simulink model "auto_pilot_upl_20240129"  (R2022b)
settings: Solver=FixedStepAuto  StartTime=0.0  StopTime=Inf  FixedStep=0.001  RelTol=1e-3  EnableMultiTasking=on
InitFcn:
  | clear mex
model workspace (MAT data in the model file):
  worldsim_instance : object (value not decoded)
values from neighbouring files (symbols this model uses):
  ACC_Adaptive_D = 0    [AutoPilot_parameters.m]    (also in ap_ini_param.mat; ap_initialModel.sldd = 0.0)
  ACC_Adaptive_I = 0    [AutoPilot_parameters.m]    (also in ap_ini_param.mat; ap_initialModel.sldd = 0.0)
  ACC_Adaptive_P = [5 7.5]    [AutoPilot_parameters.m]    (also in ap_ini_param.mat; ap_initialModel.sldd = 5.0 7.5)
  ACC_Classic_I = 5    [AutoPilot_parameters.m]    (also in ap_ini_param.mat; ap_initialModel.sldd = 5.0)
  ACC_Classic_P = 15    [AutoPilot_parameters.m]    (also in ap_ini_param.mat; ap_initialModel.sldd = 15.0)
  ACC_MaxBrake = 50    [AutoPilot_parameters.m]    (also in ap_ini_param.mat; ap_initialModel.sldd = 50.0)
  ACC_MaxThrottle = 130    [AutoPilot_parameters.m]    (also in ap_ini_param.mat = 80; ap_initialModel.sldd = 130.0)
  ACC_Module_Activity_Flag = 1    [AutoPilot_parameters.m]    (also in ap_ini_param.mat; ap_initialModel.sldd = 1.0)
  ACC_Ready_Speed = 30    [AutoPilot_parameters.m]    (also in ap_ini_param.mat; ap_initialModel.sldd = 30.0)
  ACC_SensorMaxDistance = 250    [AutoPilot_parameters.m]    (also in ap_ini_param.mat = 120; ap_initialModel.sldd = 250.0)
  ACC_Speed_Distance_control = 3    [AutoPilot_parameters.m]    (also in ap_ini_param.mat; ap_initialModel.sldd = 3.0)
  ACC_Speed_Distance_Gain = [0.1 0.15 0.2 0.25]    [AutoPilot_parameters.m]    (also in ap_ini_param.mat; ap_initialModel.sldd = 0.1 0.15 0.2 0.25)
  ADAS_Control_Mode = 1    [AutoPilot_parameters.m]    (also in ap_ini_param.mat; ap_initialModel.sldd = 1.0)
  AEB_Alarm_Freq = 5    [AutoPilot_parameters.m]    (also in ap_ini_param.mat; ap_initialModel.sldd = 5.0)
  AEB_Distance_To_Collision_Brake = 5    [AutoPilot_parameters.m]    (also in ap_ini_param.mat; ap_initialModel.sldd = 5.0)
  AEB_Freq_Hz = Sensor_Freq_worldsim/2    (= 25)    [AutoPilot_parameters.m]    (also in ap_ini_param.mat; ap_initialModel.sldd = 25.0)
  AEB_Gain = [1 1]    [AutoPilot_parameters.m]    (also in ap_ini_param.mat; ap_initialModel.sldd = 1.0 1.0)
  AEB_Gain_set = 60    [AutoPilot_parameters.m]    (also in ap_ini_param.mat; ap_initialModel.sldd = 60.0)
  AEB_Gain_set_mult = 0.03    [AutoPilot_parameters.m]    (also in ap_ini_param.mat; ap_initialModel.sldd)
  AEB_Max_Decel = [8 15]    [AutoPilot_parameters.m]    (also in ap_ini_param.mat; ap_initialModel.sldd = 8.0 15.0)
  AEB_Max_Speed = 150    [AutoPilot_parameters.m]    (also in ap_ini_param.mat = 100; ap_initialModel.sldd = 150.0)
  AEB_Min_Distance_at_Stop = 1    [AutoPilot_parameters.m]    (also in ap_ini_param.mat; ap_initialModel.sldd = 1.0)
  AEB_Module_Activity_Flag = 1    [AutoPilot_parameters.m]    (also in ap_ini_param.mat; ap_initialModel.sldd = 1.0)
  AEB_Pedestrian_type = 68    [AutoPilot_parameters.m]    (also in ap_ini_param.mat; ap_initialModel.sldd = 68.0)
  AEB_Steer_Max = 180    [AutoPilot_parameters.m]    (also in ap_ini_param.mat; ap_initialModel.sldd = 180.0)
  AP_Activity_Flag = 1    [AutoPilot_parameters.m]    (also in ap_ini_param.mat; ap_initialModel.sldd = 1.0)
  AP_D = [0.3 0.3]    [AutoPilot_parameters.m]    (also in ap_ini_param.mat; ap_initialModel.sldd = 0.3 0.3)
  AP_Dyn_Rate_Limiter_Gain = 0.1    [AutoPilot_parameters.m]    (also in ap_ini_param.mat; ap_initialModel.sldd)
  AP_Dyn_Rate_Limiter_Power = 10    [AutoPilot_parameters.m]    (also in ap_ini_param.mat; ap_initialModel.sldd = 10.0)
  AP_Error_Max = 3    [AutoPilot_parameters.m]    (also in ap_ini_param.mat; ap_initialModel.sldd = 3.0)
  AP_Freq_Hz = Sensor_Freq_worldsim    (= 50)    [AutoPilot_parameters.m]    (also in ap_ini_param.mat; ap_initialModel.sldd = 50.0)
  AP_I = [0.05 0.05]    [AutoPilot_parameters.m]    (also in ap_ini_param.mat; ap_initialModel.sldd = 0.05 0.05)
  AP_Max_Error_dydt_Disable = 0.5    [AutoPilot_parameters.m]    (also in ap_ini_param.mat; ap_initialModel.sldd)
  AP_On_Request_Time = 0.01    [AutoPilot_parameters.m]    (also in ap_ini_param.mat; ap_initialModel.sldd)
  AP_P = [0.2 0.2]    [AutoPilot_parameters.m]    (also in ap_ini_param.mat; ap_initialModel.sldd = 0.2 0.2)
  AP_Steer_Error_Max = 0.7    [AutoPilot_parameters.m]    (also in ap_ini_param.mat; ap_initialModel.sldd)
  AP_Steer_Rate_Max_radps = 1    [AutoPilot_parameters.m]    (also in ap_ini_param.mat; ap_initialModel.sldd = 1.0)
  AP_Transition_Rate = 0.5    [AutoPilot_parameters.m]    (also in ap_ini_param.mat; ap_initialModel.sldd)
  butter_a = [1 -1.9911142922 0.991153595869]    [ap_ini_param.mat]    (also in ap_initialModel.sldd = 1.0 -1.9911142922016536 0.99115359586893548)
  butter_b = [9.82591682048e-06 1.9651833641e-05 9.82591682048e-06]    [ap_ini_param.mat]    (also in ap_initialModel.sldd = 9.825916820482009E-6 1.9651833640964018E-5 9.825916820482009)
  Lane_Width = 3.7    [AutoPilot_parameters.m]    (also in ap_ini_param.mat; ap_initialModel.sldd)
  No_Target_Display_Value = 0    [AutoPilot_parameters.m]    (also in ap_ini_param.mat; ap_initialModel.sldd = 0.0)
  radar_source = 2    [AutoPilot_parameters.m]    (also in ap_ini_param.mat; ap_initialModel.sldd = 2.0)
  Sensor_Freq_worldsim = 50    [AutoPilot_parameters.m]    (also in ap_ini_param.mat; ap_initialModel.sldd = 50.0; launcher.m)
  stop_number_collisions = 10.0    [ap_initialModel.sldd]    (also in launcher.m = 10)
  stop_speed = 0.001    [ap_initialModel.sldd]    (also in launcher.m)
  stop_time = 12.0    [ap_initialModel.sldd]    (also in launcher.m = 12)
  vehicle_width = 2.2    [AutoPilot_parameters.m]    (also in ap_ini_param.mat = 1.86; ap_initialModel.sldd)
undefined symbols (not defined in the file or in its folder): blockPlatform, light_brake_center, light_brake_left, light_brake_right
libraries: simulink x82, simwbSfunlib x32, viworldsim_lib x5, slpidlib x4, simwbUDPBlocklib x1
(part 2 of 4)

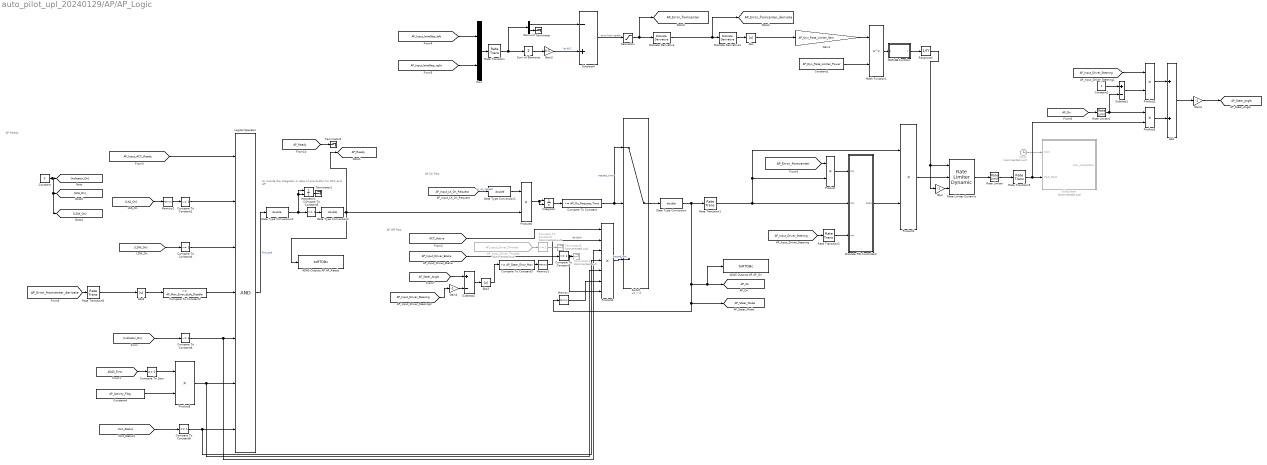
== system auto_pilot_upl_20240129/AP/AP_Logic ==
  note: to include the integrator in case of one button
      | for ACC and AP
  note: AP Off Req
  note: AP Ready
  note: AP On Req
  ADAS.Outputs.AP.AP_On : simwbSfunlib/toRTDBc  stringBlock=off  varName=ADAS.Outputs.AP.AP_On  sigDim=[1 1]  sigType=double  sampleTime=[-1 0]  maxBuffSize=1024  busName=nobus  defaultValue=0  defaultString=simwbout  hasMapping=0  ptrName=ADAS_Outputs_AP_AP_Ready  enumOrAlias=nothing
      settings: SourceProductName=SimWB MLToolkit
  ADAS.Outputs.AP.AP_Ready : simwbSfunlib/toRTDBc  stringBlock=off  varName=ADAS.Outputs.AP.AP_Ready  sigDim=[1 1]  sigType=double  sampleTime=[-1 0]  maxBuffSize=1024  busName=nobus  defaultValue=0  defaultString=simwbout  hasMapping=0  ptrName=varName  enumOrAlias=nothing
      settings: SourceProductName=SimWB MLToolkit
  AP_Input_Driver_Throttle : From  Commented=on  GotoTag=AP_Input_Driver_Throttle  TagVisibility=global
  Abs : Abs  SaturateOnIntegerOverflow=off
  Abs2 : Abs  SaturateOnIntegerOverflow=off
  Abs3 : Abs  SaturateOnIntegerOverflow=off
  Add : Sum
  Clock : Clock  Commented=on
  Compare To Constant : simulink/Logic and Bit Operations/Compare To Constant  relop=>=  const=AP_On_Request_Time  OutDataTypeStr=boolean
  Compare To Constant1 : simulink/Logic and Bit Operations/Compare To Constant  relop=~=  const=1  OutDataTypeStr=boolean
  Compare To Constant2 : simulink/Logic and Bit Operations/Compare To Constant  relop=<=  const=AP_Max_Error_dydt_Disable  OutDataTypeStr=boolean
  Compare To Constant3 : simulink/Logic and Bit Operations/Compare To Constant  relop=<=  const=AP_Steer_Error_Max  OutDataTypeStr=boolean
  Compare To Constant4 : simulink/Logic and Bit Operations/Compare To Constant  relop=~=  const=1  OutDataTypeStr=boolean
  Compare To Constant5 : simulink/Logic and Bit Operations/Compare To Constant  relop=>=  const=1  OutDataTypeStr=boolean
  Compare To Constant6 : simulink/Logic and Bit Operations/Compare To Constant  relop=~=  const=1  OutDataTypeStr=boolean
  Compare To Constant7 : simulink/Logic and Bit Operations/Compare To Constant  Commented=on  relop=<=  const=1  OutDataTypeStr=boolean
  Compare To Constant8 : simulink/Logic and Bit Operations/Compare To Constant  relop===  const=1  OutDataTypeStr=boolean
  Compare To Constant9 : simulink/Logic and Bit Operations/Compare To Constant  relop=<=  const=1  OutDataTypeStr=boolean
  Compare To Zero : simulink/Logic and Bit Operations/Compare To Zero  relop===  OutDataTypeStr=boolean
  Constant : Constant  Value=0
  Constant1 : Constant  Value=AP_Dyn_Rate_Limiter_Power
  Constant2 : Constant
  Constant4 : Constant  Value=AP_Activity_Flag
  Data Type Conversion{,1..3} (4 alike) : DataTypeConversion  OutDataTypeStr=double  SaturateOnIntegerOverflow=off  RndMeth=Floor
  Demux3 : Demux  Outputs=2
  Discrete Derivative : simulink/Discrete/Discrete Derivative  gainval=1.0  ICPrevScaledInput=0.0  OutMin=[]  OutMax=[]  OutDataType=fixdt(1, 16)  OutScaling=2^-10  DoSatur=off
  Discrete Derivative1 : simulink/Discrete/Discrete Derivative  gainval=1.0  ICPrevScaledInput=0.0  OutMin=[]  OutMax=[]  OutDataType=fixdt(1, 16)  OutScaling=2^-10  DoSatur=off
  Discrete PID Controller2 : Subsystem
  Gain : Gain  Gain=-1
  Gain1 : Gain  Gain=AP_Dyn_Rate_Limiter_Gain
  Gain2 : Gain  Gain=-1
  Gain3 : Gain  Gain=0.5
  Gain4 : Gain  Gain=-1
  Integrator : Integrator  ExternalReset=either
  Integrator1 : Integrator  ExternalReset=either
  Logical Operator : Logic  Inputs=7  AllPortsSameDT=off  OutDataTypeStr=boolean
  MATLAB Function : MATLAB Function  TreatAsAtomicUnit=on
  Math Function1 : Math  Operator=pow  SignedPower=on
  Memory : Memory
  Memory1 : Memory
  Memory2 : Memory
  Mux : Mux  Inputs=2
  Product{,1..3,5..6} (6 alike) : Product
  Product4 : Product  Inputs=7
  Rate Limiter : RateLimiter  RisingSlewLimit=AP_Steer_Rate_Max_radps  FallingSlewLimit=-AP_Steer_Rate_Max_radps  SampleTimeMode=inherited
  Rate Limiter Dynamic : simulink/Discontinuities/Rate Limiter Dynamic
  Rate Limiter1 : RateLimiter  RisingSlewLimit=AP_Transition_Rate  FallingSlewLimit=-AP_Transition_Rate  SampleTimeMode=inherited
  Rate Transition : RateTransition  OutPortSampleTime=1/AP_Freq_Hz
  Rate Transition1 : RateTransition  OutPortSampleTime=1/AP_Freq_Hz
  Rate Transition2 : RateTransition  OutPortSampleTime=1/AP_Freq_Hz
  Rate Transition5 : RateTransition  OutPortSampleTime=1/1000
  Rate Transition8 : RateTransition  OutPortSampleTime=1/1000
  Reciprocal : Product  Inputs=/  RndMeth=Zero  SaturateOnIntegerOverflow=on
  Saturation : Saturate  UpperLimit=AP_Error_Max  LowerLimit=-AP_Error_Max
  Subsystem : Subsystem  Commented=on
  Subtract1 : Sum  Inputs=+-
  Subtract2 : Sum  Inputs=+-
  Subtract4 : Sum  Inputs=-+
  Sum of Elements : Sum  Inputs=+
  Switch : Switch  Criteria=u2 > Threshold  SaturateOnIntegerOverflow=off  InputSameDT=off
  Terminator : Terminator
  Terminator1 : Terminator
  Terminator2 : Terminator
  Terminator3 : Terminator  Commented=on
  Terminator4 : Terminator  Commented=on
  tag scope: AP_Error_fromcenter=global, AP_Error_fromcenter_derivate=global, AP_On=global, AP_Ready=global, AP_Steer_Angle=global, AP_Steer_Mode=global
  wires:
  Discrete Derivative/1 -> Discrete Derivative1/1, [AP_Error_fromcenter_derivate]
  Rate Transition1/1 -> Discrete PID Controller2/2(In2), Product1/1, Product/2
  Constant1/1 -> Math Function1/2
  Math Function1/1 -> MATLAB Function/1(u)
  Discrete Derivative1/1 -> Abs/1
  Gain1/1 -> Math Function1/1
  Reciprocal/1 -> Gain/1, Rate Limiter Dynamic/1
  Abs/1 -> Gain1/1
  Gain/1 -> Rate Limiter Dynamic/3
  Rate Limiter Dynamic/1 -> Rate Limiter/1
  Product1/1 -> Rate Limiter Dynamic/2
  Clock/1 -> Subsystem/1(Clock)
  Rate Limiter/1 -> Rate Transition5/1
  Saturation/1 -> [AP_Error_fromcenter], Discrete Derivative/1
  Constant2/1 -> Subtract1/1
  Subtract1/1 -> Product2/2
  Rate Limiter1/1 -> Subtract1/2, Product3/1
  Product2/1 -> Add/1
  Product3/1 -> Add/2
  Add/1 -> Gain2/1
  Subtract2/1 -> Abs3/1
  [AP_Input_LK_On_Request] -> Data Type Conversion1/1  "LK_on_request"
  Switch/1 -> Data Type Conversion/1
  Product4/1 -> Switch/3  "second_and"
  Data Type Conversion/1 -> Memory/1, [AP_Steer_Mode], ADAS.Outputs.AP.AP_On/1, [AP_On], Rate Transition1/1
  Data Type Conversion1/1 -> Product6/1
  Rate Transition8/1 -> Abs2/1
  Abs2/1 -> Compare To Constant2/1
  Compare To Constant2/1 -> Logical Operator/4
  Abs3/1 -> Compare To Constant3/1
  Compare To Constant3/1 -> Memory1/1
  [LDW_On] -> Compare To Constant4/1
  Compare To Constant4/1 -> Logical Operator/3
  Memory1/1 -> Product4/2  "de-latch"
  [LKA_On] -> Memory2/1
  Memory2/1 -> Compare To Constant1/1
  Integrator/1 -> Compare To Constant/1
  Product6/1 -> Integrator/1, Integrator/2
  Compare To Constant1/1 -> Logical Operator/2
  Logical Operator/1 -> Data Type Conversion3/1  "first_and"
  Compare To Constant/1 -> Switch/1, Switch/2  "request_time"
  Data Type Conversion2/1 -> Product6/2, ADAS.Outputs.AP.AP_Ready/1, [AP_Ready]
  Data Type Conversion3/1 -> Integrator1/1, Integrator1/2, Compare To Constant5/1
  Compare To Constant5/1 -> Data Type Conversion2/1
  [Indicator_On] -> Compare To Constant6/1
  Compare To Constant6/1 -> Product4/3, Logical Operator/5
  Rate Transition/1 -> Demux3/1, Sum of Elements/1
  Sum of Elements/1 -> Gain3/1
  Gain3/1 -> Subtract4/2  "(a+b)/2"
  Demux3/2 -> Terminator/1
  Demux3/1 -> Subtract4/1
  Subtract4/1 -> Saturation/1  "error from center"
  [ADAS_Error] -> Compare To Zero/1
  Constant4/1 -> Product5/2
  Compare To Zero/1 -> Product5/1
  Product5/1 -> Logical Operator/6, Product4/5
  [Vicrt_Status] -> Compare To Constant8/1
  Compare To Constant8/1 -> Product4/4, Logical Operator/7
  [AP_Input_Driver_Steering] -> Rate Transition2/1
  Product/1 -> Discrete PID Controller2/1(In1)
  Rate Transition2/1 -> Discrete PID Controller2/3(In4)
  Discrete PID Controller2/1(Out1) -> Product1/2
  Rate Transition5/1 -> Product3/2, Subsystem/2(Input_Signal)
  [AP_Input_ACC_Ready] -> Logical Operator/1
  AP_Input_Driver_Throttle/1 -> Compare To Constant7/1
  Compare To Constant9/1 -> Product4/7, Terminator4/1
  [AP_Input_Driver_Brake] -> Compare To Constant9/1
  Compare To Constant7/1 -> Terminator3/1
  [ACC_Active] -> Product4/1
  Integrator1/1 -> Terminator1/1
  Mux/1 -> Rate Transition/1
  [AP_Input_laneGap_left] -> Mux/1
  [AP_Input_laneGap_right] -> Mux/2
  [AP_Error_fromcenter_derivate] -> Rate Transition8/1
  [AP_Input_Driver_Steering] -> Product2/1
  [AP_Input_Driver_Steering] -> Gain4/1
  [AP_Steer_Angle] -> Subtract2/1
  [AP_On] -> Rate Limiter1/1
  [AP_Error_fromcenter] -> Product/1
  Gain2/1 -> [AP_Steer_Angle]
  Memory/1 -> Product4/6
  Gain4/1 -> Subtract2/2
  Constant/1 -> [LDW_On], [LKA_On], [Indicator_On]
  [AP_Ready] -> Terminator2/1
  MATLAB Function/1(y) -> Reciprocal/1

== system auto_pilot_upl_20240129/AP/AP_Outputs ==
  Terminator : Terminator
  tag scope: AP_Output_Steer_Angle=global, AP_Output_Steer_Torque=global
  wires:
  [AP_Steer_Mode] -> [AP_Output_Steer_Torque]
  [AP_Steer_Angle] -> [AP_Output_Steer_Angle]
  [AP_Output_Steer_Torque] -> Terminator/1

== system auto_pilot_upl_20240129/INPUT/Inputs for CRT ==
  Clutch_manager : Subsystem
  Constant : Constant  Value=0
  Constant1 : Constant
  tag scope: brake_demand=global, clutch_demand=global, gear_demand=global, steering_angle_demand=global, steering_torque_demand=global, throttle_demand=global
  wires:
  [ACC_Output_Brake] -> [brake_demand]
  Constant/1 -> [steering_torque_demand]
  [AP_Output_Steer_Angle] -> [steering_angle_demand]
  Clutch_manager/1(clutch) -> [clutch_demand]
  [ACC_Output_Throttle] -> [throttle_demand]
  [ACC_Output_Throttle] -> Clutch_manager/1(throttle)
  Constant1/1 -> [gear_demand]

== system auto_pilot_upl_20240129/OUTPUT/VI-CarRealTime_Outputs ==
  Gain : Gain  Gain=1/2
  Log_bus : BusSelector  OutputSignals=VI_CarRealTime:Outputs:chassis_velocities:longitudinal,VI_CarRealTime:Outputs:driver_demands:steering,VI_CarRealTime:Outputs:Wheel:Spindle_Steer:L1,VI_CarRealTime:Outputs:Wheel:Spindle_Steer:R1,VI_CarRealTime:Outputs:driver_demands:throttle,VI_CarRealTime:Outputs:driver_demands:brake,VI_CarRealTime:Outputs:chassis_accelerations:longitudinal,VI_CarRealTime:Outputs:chassis_accelerations:lateral,VI_CarRealTime:Outputs:Steering_System:DriveSim_Steering_Feedback_Torque  OutputAsBus=on
  Scope : Scope  NumInputPorts=2
  Sum : Sum
  Terminator : Terminator
  internal_bus : BusSelector  OutputSignals=VI_CarRealTime:Outputs:chassis_velocities:longitudinal,VI_CarRealTime:Outputs:driver_demands:steering,VI_CarRealTime:Outputs:Wheel:Spindle_Steer:L1,VI_CarRealTime:Outputs:Wheel:Spindle_Steer:R1,VI_CarRealTime:Outputs:driver_demands:throttle,VI_CarRealTime:Outputs:driver_demands:brake,VI_CarRealTime:Outputs:chassis_accelerations:longitudinal,VI_CarRealTime:Outputs:chassis_accelerations:lateral,VI_CarRealTime:Outputs:Steering_System:DriveSim_Steering_Feedback_Torque
  tag scope: Driver_Brake=global, Driver_Steering=global, Driver_Throttle=global, Front_Axle_Steer=global, Lateral_Accelerations=global, Longitudinal_Accelerations=global, Steering_feedback_torque=global, Vehicle_Speed=global
  wires:
  internal_bus/9 -> [Steering_feedback_torque]  "<VI_CarRealTime:Outputs:Steering_System:DriveSim_Steering_Feedback_Torque>"
  internal_bus/8 -> [Lateral_Accelerations]  "<VI_CarRealTime:Outputs:chassis_accelerations:lateral>"
  internal_bus/7 -> [Longitudinal_Accelerations]  "<VI_CarRealTime:Outputs:chassis_accelerations:longitudinal>"
  internal_bus/6 -> [Driver_Brake]  "<VI_CarRealTime:Outputs:driver_demands:brake>"
  internal_bus/5 -> [Driver_Throttle]  "<VI_CarRealTime:Outputs:driver_demands:throttle>"
  Gain/1 -> [Front_Axle_Steer]
  Sum/1 -> Gain/1
  internal_bus/4 -> Sum/2  "<VI_CarRealTime:Outputs:Wheel:Spindle_Steer:R1>"
  internal_bus/3 -> Sum/1  "<VI_CarRealTime:Outputs:Wheel:Spindle_Steer:L1>"
  [Vehicle_outputs] -> internal_bus/1, Log_bus/1
  internal_bus/2 -> [Driver_Steering], Scope/2  "<VI_CarRealTime:Outputs:driver_demands:steering>"
  Log_bus/1 -> Terminator/1  "VI_CarRealTime_selection"
  internal_bus/1 -> [Vehicle_Speed], Scope/1  "<VI_CarRealTime:Outputs:chassis_velocities:longitudinal>"

== system auto_pilot_upl_20240129/OUTPUT/VI-CarRealTime_Outputs2 ==
  Constant : Constant  Value=0
  Gain : Gain  Gain=1/2
  Log_Bus_Creator : BusCreator  Inputs=9
  Log_bus : BusSelector  OutputSignals=VI_CarRealTime:Outputs:chassis_velocities:longitudinal,VI_CarRealTime:Outputs:driver_demands:steering,VI_CarRealTime:Outputs:Wheel:Spindle_Steer:L1,VI_CarRealTime:Outputs:Wheel:Spindle_Steer:R1,VI_CarRealTime:Outputs:driver_demands:throttle,VI_CarRealTime:Outputs:driver_demands:brake,VI_CarRealTime:Outputs:chassis_accelerations:longitudinal,VI_CarRealTime:Outputs:chassis_accelerations:lateral,VI_CarRealTime:Outputs:Steering_System:DriveSim_Steering_Feedback_Torque  OutputAsBus=on
  Scope : Scope  NumInputPorts=2
  Sum : Sum
  Terminator : Terminator
  Terminator1 : Terminator
  VI_CarRealTime.Outputs.Steering_System.DriveSim_Steering_Feedback_Torque : simwbSfunlib/fromRTDBm  varName=VI_CarRealTime.Outputs.Steering_System.DriveSim_Steering_Feedback_Torque  sigDim=[1 1]  sigType=double  sampleTime=[-1 0]  defaultValue=0  hasMapping=0  ptrName=VI_CarRealTime_Outputs_chassis_accelerations_lateral  enumOrAlias=nothing
      settings: SourceProductName=SimWB MLToolkit
  VI_CarRealTime.Outputs.Wheel.Spindle_Steer.L1 : simwbSfunlib/fromRTDBm  varName=VI_CarRealTime.Outputs.Wheel.Spindle_Steer.L1  sigDim=[1 1]  sigType=double  sampleTime=[-1 0]  defaultValue=0  hasMapping=0  ptrName=VI_CarRealTime_Outputs_Wheel_Spindle_Steer_L1  enumOrAlias=nothing
      settings: SourceProductName=SimWB MLToolkit
  VI_CarRealTime.Outputs.Wheel.Spindle_Steer.R1 : simwbSfunlib/fromRTDBm  varName=VI_CarRealTime.Outputs.Wheel.Spindle_Steer.R1  sigDim=[1 1]  sigType=double  sampleTime=[-1 0]  defaultValue=0  hasMapping=0  ptrName=VI_CarRealTime_Outputs_Wheel_Spindle_Steer_R1  enumOrAlias=nothing
      settings: SourceProductName=SimWB MLToolkit
  VI_CarRealTime.Outputs.chassis_accelerations.lateral : simwbSfunlib/fromRTDBm  varName=VI_CarRealTime.Outputs.chassis_accelerations.lateral  sigDim=[1 1]  sigType=double  sampleTime=[-1 0]  defaultValue=0  hasMapping=0  ptrName=VI_CarRealTime_Outputs_chassis_accelerations_longitudinal  enumOrAlias=nothing
      settings: SourceProductName=SimWB MLToolkit
  VI_CarRealTime.Outputs.chassis_accelerations.longitudinal : simwbSfunlib/fromRTDBm  varName=VI_CarRealTime.Outputs.chassis_accelerations.longitudinal  sigDim=[1 1]  sigType=double  sampleTime=[-1 0]  defaultValue=0  hasMapping=0  ptrName=VI_CarRealTime_Outputs_chassis_velocities_longitudinal  enumOrAlias=nothing
      settings: SourceProductName=SimWB MLToolkit
  VI_CarRealTime.Outputs.chassis_velocities.longitudinal : simwbSfunlib/fromRTDBm  varName=VI_CarRealTime.Outputs.chassis_velocities.longitudinal  sigDim=[1 1]  sigType=double  sampleTime=[-1 0]  defaultValue=0  hasMapping=0  ptrName=VI_CarRealTime_Outputs_chassis_velocities_longitudinal  enumOrAlias=nothing
      settings: SourceProductName=SimWB MLToolkit
  VI_CarRealTime.Outputs.driver_demands.brake : simwbSfunlib/fromRTDBm  varName=VI_CarRealTime.Outputs.driver_demands.brake  sigDim=[1 1]  sigType=double  sampleTime=[-1 0]  defaultValue=0  hasMapping=0  ptrName=VI_CarRealTime_Outputs_driver_demands_throttle  enumOrAlias=nothing
      settings: SourceProductName=SimWB MLToolkit
  VI_CarRealTime.Outputs.driver_demands.steering : simwbSfunlib/fromRTDBm  varName=VI_CarRealTime.Outputs.driver_demands.steering  sigDim=[1 1]  sigType=double  sampleTime=[-1 0]  defaultValue=0  hasMapping=0  ptrName=VI_CarRealTime_Outputs_chassis_velocities_longitudinal  enumOrAlias=nothing
      settings: SourceProductName=SimWB MLToolkit
  VI_CarRealTime.Outputs.driver_demands.throttle : simwbSfunlib/fromRTDBm  varName=VI_CarRealTime.Outputs.driver_demands.throttle  sigDim=[1 1]  sigType=double  sampleTime=[-1 0]  defaultValue=0  hasMapping=0  ptrName=VI_CarRealTime_Outputs_driver_demands_steering  enumOrAlias=nothing
      settings: SourceProductName=SimWB MLToolkit
  tag scope: Driver_Brake=global, Driver_Steering=global, Driver_Throttle=global, Front_Axle_Steer=global, Lateral_Accelerations=global, Longitudinal_Accelerations=global, Steering_feedback_torque=global, Vehicle_Speed=global
  wires:
  ? -> Scope/1, [Vehicle_Speed]
  Log_bus/1 -> Terminator/1  "VI_CarRealTime_selection"
  ? -> Scope/2, [Driver_Steering]
  ? -> Sum/1
  ? -> Sum/2
  Sum/1 -> Gain/1
  Gain/1 -> [Front_Axle_Steer]
  ? -> [Driver_Throttle]
  Constant/1 -> [Driver_Brake]
  ? -> Terminator1/1
  ? -> [Longitudinal_Accelerations]
  ? -> [Lateral_Accelerations]
  ? -> [Steering_feedback_torque]
  VI_CarRealTime.Outputs.driver_demands.brake/1 -> Log_Bus_Creator/6  "VI_CarRealTime.Outputs.driver_demands.brake"
  VI_CarRealTime.Outputs.Wheel.Spindle_Steer.L1/1 -> Log_Bus_Creator/3  "VI_CarRealTime.Outputs.Wheel.Spindle_Steer.L1"
  VI_CarRealTime.Outputs.chassis_accelerations.lateral/1 -> Log_Bus_Creator/8  "VI_CarRealTime.Outputs.chassis_accelerations.lateral"
  VI_CarRealTime.Outputs.Steering_System.DriveSim_Steering_Feedback_Torque/1 -> Log_Bus_Creator/9  "VI_CarRealTime.Outputs.Steering_System.DriveSim_Steering_Feedback_Torque"
  VI_CarRealTime.Outputs.chassis_accelerations.longitudinal/1 -> Log_Bus_Creator/7  "VI_CarRealTime.Outputs.chassis_accelerations.longitudinal"
  VI_CarRealTime.Outputs.driver_demands.steering/1 -> Log_Bus_Creator/2  "VI_CarRealTime.Outputs.driver_demands.steering"
  VI_CarRealTime.Outputs.Wheel.Spindle_Steer.R1/1 -> Log_Bus_Creator/4  "VI_CarRealTime.Outputs.Wheel.Spindle_Steer.R1"
  VI_CarRealTime.Outputs.driver_demands.throttle/1 -> Log_Bus_Creator/5  "VI_CarRealTime.Outputs.driver_demands.throttle"
  VI_CarRealTime.Outputs.chassis_velocities.longitudinal/1 -> Log_Bus_Creator/1  "VI_CarRealTime.Outputs.chassis_velocities.longitudinal"
  Log_Bus_Creator/1 -> Log_bus/1

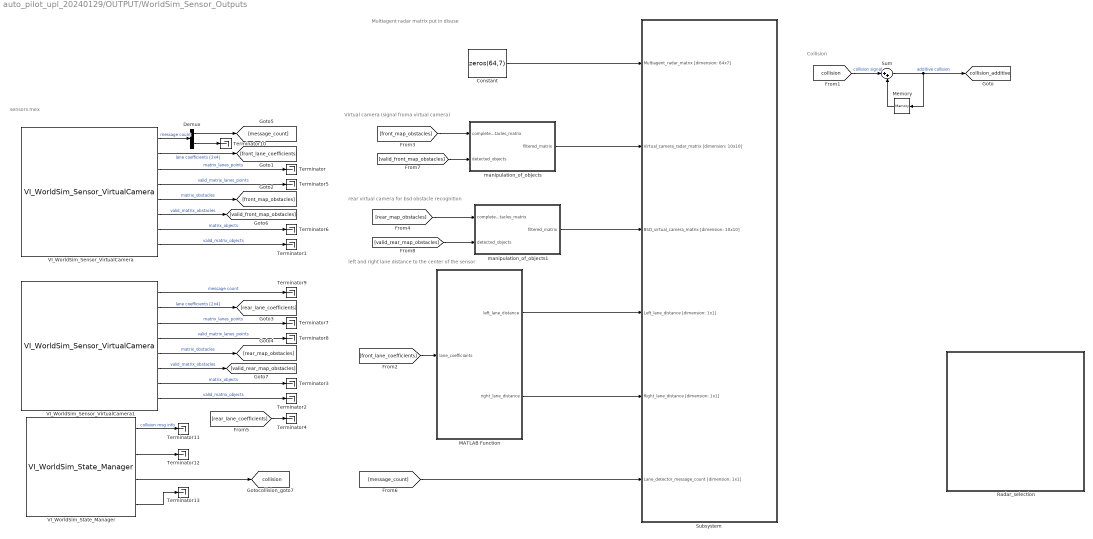
== system auto_pilot_upl_20240129/OUTPUT/WorldSim_Sensor_Outputs ==
  note: Collision
  note: left and right lane distance to the center of the sensor
  note: Virtual camera (signal froma virtual camera)
  note: Multiagent radar matrix
      | put in disuse
  note: rear virtual camera for bsd obstacle recognition
  note: sensors mex
  Constant : Constant  Value=zeros(64,7)
  Demux : Demux  Outputs=2
  MATLAB Function : MATLAB Function  TreatAsAtomicUnit=on
  Memory : Memory  InheritSampleTime=on
  Radar_selection : Subsystem
  Subsystem : Subsystem
  Sum : Sum  Inputs=|++
  Terminator{,1..13} (14 alike) : Terminator
  VI_WorldSim_Sensor_VirtualCamera : viworldsim_lib/VI-WorldSim Sensors/VI_WorldSim_Sensor_VirtualCamera  worldsim_endpoint_ip=worldsim_instance.endpoint_ip  worldsim_endpoint_port=worldsim_instance.endpoint_port  worldsim_car_name='ego'  worldsim_sensor_name='Front_VirtualCam'  max_lanes=10  max_obstacles=10  worldsim_verbose=off
  VI_WorldSim_Sensor_VirtualCamera1 : viworldsim_lib/VI-WorldSim Sensors/VI_WorldSim_Sensor_VirtualCamera  worldsim_endpoint_ip=worldsim_instance.endpoint_ip  worldsim_endpoint_port=worldsim_instance.endpoint_port  worldsim_car_name='ego'  worldsim_sensor_name='Rear_VirtualCam'  max_lanes=10  max_obstacles=10  worldsim_verbose=off
  VI_WorldSim_State_Manager : viworldsim_lib/VI-WorldSim Sensors/VI_WorldSim_State_Manager  worldsim_endpoint_ip=worldsim_instance.endpoint_ip  worldsim_endpoint_port=worldsim_instance.endpoint_port  worldsim_car_name='ego'  worldsim_verbose=off
  manipulation_of_objects : MATLAB Function  TreatAsAtomicUnit=on
  manipulation_of_objects1 : MATLAB Function  TreatAsAtomicUnit=on
  tag scope: collision=global, collision_additive=global
  wires:
  Sum/1 -> Memory/1, [collision_additive]  "additive collision"
  [collision] -> Sum/1  "collision signal"
  Memory/1 -> Sum/2
  MATLAB Function/1(left_lane_distance) -> Subsystem/4(Left_lane_distance [dimension: 1x1])
  [message_count] -> Subsystem/6(Lane_detector_message_count [dimension: 1x1])
  manipulation_of_objects1/1(filtered_matrix) -> Subsystem/3(BSD_virtual_camera_matrix [dimension: 10x10])
  manipulation_of_objects/1(filtered_matrix) -> Subsystem/2(Virtual_camera_radar_matrix [dimension: 10x10])
  Constant/1 -> Subsystem/1(Multiagent_radar_matrix [dimension: 64x7])
  [valid_rear_map_obstacles] -> manipulation_of_objects1/2(detected_objects)
  MATLAB Function/2(right_lane_distance) -> Subsystem/5(Right_lane_distance [dimension: 1x1])
  [front_lane_coefficients] -> MATLAB Function/1(lane_coefficiants)
  [rear_map_obstacles] -> manipulation_of_objects1/1(complete_obstacles_matrix)
  [valid_front_map_obstacles] -> manipulation_of_objects/2(detected_objects)
  [front_map_obstacles] -> manipulation_of_objects/1(complete_obstacles_matrix)
  VI_WorldSim_Sensor_VirtualCamera/1 -> Demux/1  "message count"
  VI_WorldSim_State_Manager/1 -> Terminator11/1  "collision msg info"
  VI_WorldSim_Sensor_VirtualCamera/8 -> Terminator1/1  "valid_matrix_objects"
  VI_WorldSim_Sensor_VirtualCamera/5 -> [front_map_obstacles]  "matrix_obstacles"
  VI_WorldSim_Sensor_VirtualCamera/4 -> Terminator5/1  "valid_matrix_lanes_points"
  VI_WorldSim_Sensor_VirtualCamera/6 -> [valid_front_map_obstacles]  "valid_matrix_obstacles"
  VI_WorldSim_Sensor_VirtualCamera1/2 -> [rear_lane_coefficients]  "lane coefficients [2x4]"
  VI_WorldSim_Sensor_VirtualCamera/3 -> Terminator/1  "matrix_lanes_points"
  VI_WorldSim_Sensor_VirtualCamera1/1 -> Terminator9/1  "message count"
  VI_WorldSim_Sensor_VirtualCamera1/7 -> Terminator3/1  "matrix_objects"
  VI_WorldSim_Sensor_VirtualCamera1/8 -> Terminator2/1  "valid_matrix_objects"
  VI_WorldSim_Sensor_VirtualCamera/7 -> Terminator6/1  "matrix_objects"
  VI_WorldSim_Sensor_VirtualCamera/2 -> [front_lane_coefficients]  "lane coefficients [2x4]"
  VI_WorldSim_Sensor_VirtualCamera1/4 -> Terminator8/1  "valid_matrix_lanes_points"
  VI_WorldSim_State_Manager/3 -> [collision]
  VI_WorldSim_Sensor_VirtualCamera1/3 -> Terminator7/1  "matrix_lanes_points"
  [rear_lane_coefficients] -> Terminator4/1
  Demux/2 -> Terminator10/1
  VI_WorldSim_Sensor_VirtualCamera1/5 -> [rear_map_obstacles]  "matrix_obstacles"
  VI_WorldSim_Sensor_VirtualCamera1/6 -> [valid_rear_map_obstacles]  "valid_matrix_obstacles"
  Demux/1 -> [message_count]
  VI_WorldSim_State_Manager/2 -> Terminator12/1
  VI_WorldSim_State_Manager/4 -> Terminator13/1

== system auto_pilot_upl_20240129/OUTPUT/rough data reporting ==
  Cast To Double : DataTypeConversion  OutDataTypeStr=double  SaturateOnIntegerOverflow=off  RndMeth=Floor
  Cast To Double1 : DataTypeConversion  OutDataTypeStr=double  SaturateOnIntegerOverflow=off  RndMeth=Floor
  Clock : Clock
  Compare To Constant : simulink/Logic and Bit Operations/Compare To Constant  relop=<=  const=0.0  OutDataTypeStr=boolean
  Compare To Constant1 : simulink/Logic and Bit Operations/Compare To Constant  relop=<=  const=0.0  OutDataTypeStr=boolean
  Compare To Constant2 : simulink/Logic and Bit Operations/Compare To Constant  relop=>  const=0.1  OutDataTypeStr=boolean
  Constant : Constant  Value=0
  Mux : Mux  Inputs=2
  Product : Product
  Scope LDW_Steering_Torque_in_out : Scope
  Sum1 : Sum
  To Workspace : ToWorkspace  VariableName=number_collision  SampleTime=-1
      settings: Save2DSignal=2-D array (concatenate along first dimension)
  To Workspace1 : ToWorkspace  VariableName=longitudinal_accelerations  SampleTime=-1
      settings: Save2DSignal=2-D array (concatenate along first dimension)
  To Workspace2 : ToWorkspace  VariableName=lateral_accelerations  SampleTime=-1
      settings: Save2DSignal=2-D array (concatenate along first dimension)
  To Workspace3 : ToWorkspace  VariableName=crossed_lanes  SampleTime=-1
      settings: Save2DSignal=2-D array (concatenate along first dimension)
  wires:
  Clock/1 -> Compare To Constant2/1
  Compare To Constant1/1 -> Cast To Double1/1
  [Lateral_Accelerations] -> To Workspace2/1
  [LaneGap_right_ws] -> Compare To Constant1/1
  Cast To Double/1 -> Sum1/1
  Compare To Constant2/1 -> Product/2
  [collision_additive] -> To Workspace/1
  Compare To Constant/1 -> Cast To Double/1
  [Longitudinal_Accelerations] -> To Workspace1/1
  [LaneGap_left_ws] -> Compare To Constant/1
  Product/1 -> To Workspace3/1
  Cast To Double1/1 -> Sum1/2
  Sum1/1 -> Product/1
  [Steering_feedback_torque] -> Mux/2
  [LDW_Steering_Torque] -> Mux/1
  Mux/1 -> Scope LDW_Steering_Torque_in_out/1  "LDW_Steering_Torque_in_out"
  Constant/1 -> [LDW_Steering_Torque]

== system auto_pilot_upl_20240129/VI-WorldSim Lights Manager/Lights ==
  light_brake_left : Inport
  light_brake_right : Inport  Port=2
  light_brake_center : Inport  Port=3
  Bus Selector : BusSelector  OutputSignals=light_low_beam_left,light_low_beam_right,light_high_beam_left,light_high_beam_right,light_indicator_left,light_indicator_right,light_fog_left,light_fog_right,light_tail_left,light_tail_right,light_brake_left,light_brake_right,light_brake_center,light_reverse,light_daytime
  Default Lights Bus : Subsystem
  LightsBusAssignment : BusAssignment  AssignedSignals=light_brake_left,light_brake_right,light_brake_center
  Mux : Mux  Inputs=15
  Out1 : Outport  VectorParamsAs1DForOutWhenUnconnected=off
  wires:
  LightsBusAssignment/1 -> Bus Selector/1
  Bus Selector/5 -> Mux/5  "<light_indicator_left>"
  Default Lights Bus/1(Out1) -> LightsBusAssignment/1
  Bus Selector/11 -> Mux/11  "<light_brake_left>"
  Bus Selector/10 -> Mux/10  "<light_tail_right>"
  Bus Selector/2 -> Mux/2  "<light_low_beam_right>"
  Bus Selector/9 -> Mux/9  "<light_tail_left>"
  Bus Selector/12 -> Mux/12  "<light_brake_right>"
  Mux/1 -> Out1/1
  Bus Selector/8 -> Mux/8  "<light_fog_right>"
  Bus Selector/14 -> Mux/14  "<light_reverse>"
  Bus Selector/4 -> Mux/4  "<light_high_beam_right>"
  Bus Selector/3 -> Mux/3  "<light_high_beam_left>"
  Bus Selector/15 -> Mux/15  "<light_daytime>"
  Bus Selector/13 -> Mux/13  "<light_brake_center>"
  Bus Selector/6 -> Mux/6  "<light_indicator_right>"
  Bus Selector/1 -> Mux/1  "<light_low_beam_left>"
  Bus Selector/7 -> Mux/7  "<light_fog_left>"
  light_brake_left/1 -> LightsBusAssignment/2
  light_brake_right/1 -> LightsBusAssignment/3
  light_brake_center/1 -> LightsBusAssignment/4

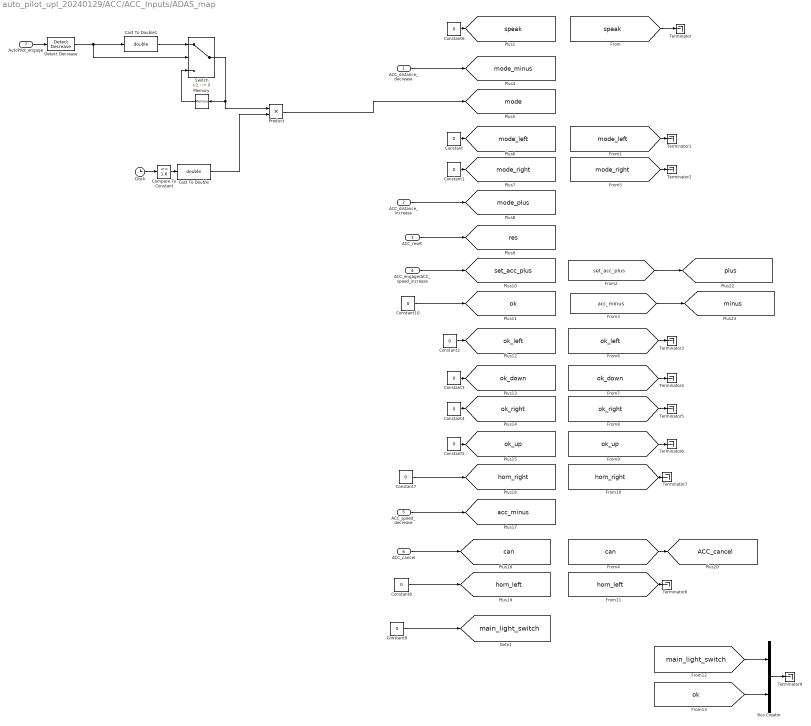
== system auto_pilot_upl_20240129/ACC/ACC_Inputs/ADAS_map ==
  ACC_distance_decrease : Inport
  ACC_distance_increase : Inport  Port=2
  ACC_reset : Inport  Port=3
  ACC_engage/ACC_speed_increase : Inport  Port=4
  ACC_speed_decrease : Inport  Port=5
  ACC_cancel : Inport  Port=6
  AutoPilot_engage : Inport  Port=7
  Bus Creator : BusCreator  Inputs=2
  Cast To Double : DataTypeConversion  OutDataTypeStr=double  SaturateOnIntegerOverflow=off  RndMeth=Floor
  Cast To Double1 : DataTypeConversion  OutDataTypeStr=double  SaturateOnIntegerOverflow=off  RndMeth=Floor
  Clock : Clock
  Compare To Constant : simulink/Logic and Bit Operations/Compare To Constant  relop=<=  const=1.6  OutDataTypeStr=boolean
  Constant{,1..10} (11 alike) : Constant  Value=0
  Detect Decrease : simulink/Logic and Bit Operations/Detect Decrease  vinit=0.0  OutDataTypeStr=boolean
  Memory : Memory  InheritSampleTime=on
  Product : Product
  Switch : Switch  Criteria=u2 ~= 0  SaturateOnIntegerOverflow=off  InputSameDT=off
  Terminator{,1..9} (10 alike) : Terminator
  tag scope: ACC_cancel=global, acc_minus=global, can=global, horn_left=global, horn_right=global, main_light_switch=global, minus=global, mode=global, mode_left=global, mode_minus=global, mode_plus=global, mode_right=global, ok=global, ok_down=global, ok_left=global, ok_right=global, ok_up=global, plus=global, res=global, set_acc_plus=global, speak=global
  wires:
  [set_acc_plus] -> [plus]
  ACC_speed_decrease/1 -> [acc_minus]
  Constant10/1 -> [ok]
  Constant8/1 -> [horn_left]
  [acc_minus] -> [minus]
  ACC_engage/ACC_speed_increase/1 -> [set_acc_plus]
  ACC_reset/1 -> [res]
  ACC_cancel/1 -> [can]
  ACC_distance_increase/1 -> [mode_plus]
  ACC_distance_decrease/1 -> [mode_minus]
  Constant7/1 -> [horn_right]
  Constant6/1 -> [speak]
  [can] -> [ACC_cancel]
  Constant9/1 -> [main_light_switch]
  Constant/1 -> [mode_left]
  Constant1/1 -> [mode_right]
  Constant2/1 -> [ok_left]
  Constant3/1 -> [ok_down]
  Constant4/1 -> [ok_right]
  Constant5/1 -> [ok_up]
  [speak] -> Terminator/1
  [mode_left] -> Terminator1/1
  [mode_right] -> Terminator2/1
  [ok_left] -> Terminator3/1
  [ok_down] -> Terminator4/1
  [ok_right] -> Terminator5/1
  [ok_up] -> Terminator6/1
  [horn_right] -> Terminator7/1
  [horn_left] -> Terminator8/1
  AutoPilot_engage/1 -> Detect Decrease/1
  Switch/1 -> Product/1, Memory/1
  Memory/1 -> Switch/3
  Clock/1 -> Compare To Constant/1
  Compare To Constant/1 -> Cast To Double/1
  Cast To Double/1 -> Product/2
  Product/1 -> [mode]
  [main_light_switch] -> Bus Creator/1
  [ok] -> Bus Creator/2
  Bus Creator/1 -> Terminator9/1
  Detect Decrease/1 -> Switch/2, Cast To Double1/1
  Cast To Double1/1 -> Switch/1

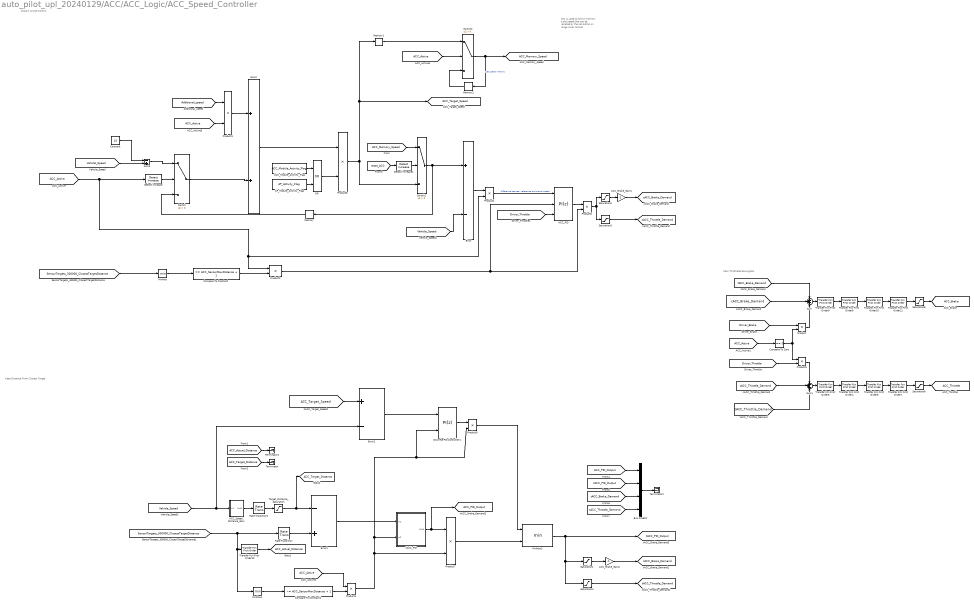
== system auto_pilot_upl_20240129/ACC/ACC_Logic/ACC_Speed_Controller ==
  note: this is used to hold in memory a set speed that can be recalled by the res button on range rover cockpit
  note: Pass Throttle/Brake signals
  note: Keep Distance From Closest Target
  note: Classic Cruise Control
  ACC_Brake_Gain1 : Gain  Gain=-1
  ACC_Brake_Gain2 : Gain  Gain=-1
  ACC_Module_Activity_Flag : Constant  Value=ACC_Module_Activity_Flag
  ACC_PID : slpidlib/PID Controller  Controller=PI  Form=Parallel  TimeDomain=Discrete-time  UseExternalTs=off  SampleTime=-1  IntegratorMethod=Forward Euler  FilterMethod=Forward Euler  ControllerParametersSource=internal  P=ACC_Classic_P  I=ACC_Classic_I  UseKiTs=off  D=0  N=100  UseFilter=on  TunerSelectOption=Transfer Function Based (PID Tuner App)  InitialConditionSource=external  InitialConditionForIntegrator=0  InitialConditionForFilter=0  DifferentiatorICPrevScaledInput=0  ExternalReset=either  TrackingMode=off  Kt=1  LimitOutput=on  SatLimitsSource=internal  UpperSaturationLimit=ACC_MaxThrottle  LowerSaturationLimit=-ACC_MaxBrake  LinearizeAsGain=off  AntiWindupMode=back-calculation  Kb=1  LimitIntegrator=off  UpperIntegratorSaturationLimit=inf  LowerIntegratorSaturationLimit=-inf  POutMin=[]  POutMax=[]  IOutMin=[]  IOutMax=[]  DOutMin=[]  DOutMax=[]  NOutMin=[]  NOutMax=[]  SumOutMin=[]  SumOutMax=[]  SaturationOutMin=[]  SaturationOutMax=[]  PParamMin=[]  PParamMax=[]  IParamMin=[]  IParamMax=[]  DParamMin=[]  DParamMax=[]  NParamMin=[]  NParamMax=[]  KbParamMin=[]  KbParamMax=[]  KtParamMin=[]  KtParamMax=[]  KbOutMin=[]  KbOutMax=[]  KtOutMin=[]  KtOutMax=[]  IntegratorOutMin=[]  IntegratorOutMax=[]  FilterOutMin=[]  FilterOutMax=[]  SumI1OutMin=[]  SumI1OutMax=[]  SumI2OutMin=[]  SumI2OutMax=[]  SumI3OutMin=[]  SumI3OutMax=[]  SumI4OutMin=[]  SumI4OutMax=[]  SumDOutMin=[]  SumDOutMax=[]  DifferentiatorOutMin=[]  DifferentiatorOutMax=[]  FilterDiffOutCoefMin=[]  FilterDiffOutCoefMax=[]  ReciprocalOutMin=[]  ReciprocalOutMax=[]  SumDenOutMin=[]  SumDenOutMax=[]  SumNumOutMin=[]  SumNumOutMax=[]  DivideOutMin=[]  DivideOutMax=[]  UdiffTsProdOutMin=[]  UdiffTsProdOutMax=[]  NTsProdOutMin=[]  NTsProdOutMax=[]  UintegralTsProdOutMin=[]  UintegralTsProdOutMax=[]  UngainTsProdOutMin=[]  UngainTsProdOutMax=[]  ClampingZeroOutDataTypeStr=Inherit: Inherit via back propagation  ClampingZeroOutMin=[]  ClampingZeroOutMax=[]  FilterDenConstantOutDataTypeStr=Inherit: Inherit via back propagation  FilterDenConstantOutMin=[]  FilterDenConstantOutMax=[]  PCopyOutDataTypeStr=Inherit: Inherit via back propagation  PCopyOutMin=[]  PCopyOutMax=[]  NCopyOutDataTypeStr=Inherit: Inherit via back propagation  NCopyOutMin=[]  NCopyOutMax=[]  IntegratorContinuousStateAttributes=''  IntegratorStateMustResolveToSignalObject=off  IntegratorRTWStateStorageClass=Auto  FilterContinuousStateAttributes=''  FilterStateMustResolveToSignalObject=off  FilterRTWStateStorageClass=Auto  ParallelPVariant=InternalParameters  IdealPVariant=Disabled  IVariant=InternalParameters  DVariant=Disabled  IntegratorVariant=Discrete  SatVariant=Enabled  AWVariant=BackCalculation  PCopyVariant=Disabled  TRVariant=Disabled  FdbkBlocksVariant=Forward  IdealPFdbkVariant=Disabled  SatFdbkVariant=Disabled  DerivativeFilterVariant=Disabled  NVariant=Disabled  NCopyVariant=Disabled_SignalSpec  FilterICVariant=Disabled  IntegratorICVariant=ExternalICs  ExternalResetVariant=ExternalReset  TRSumVariant=Passthrough  SumFdbkVariant=Disabled  SumVariant=Sum_PI  TsampFilterVariant=InternalTs  TsampNgainVariant=Passthrough  TsampIntegralVariant=Passthrough  ExternalSaturationOutDataTypeStr=Inherit: Same as second input
  ACC_Speed_Distance_Gain : Subsystem
  AP_Module_Activity_Flag : Constant  Value=AP_Activity_Flag
  Bus Creator : BusCreator  Inputs=4
  Compare To Constant : simulink/Logic and Bit Operations/Compare To Constant  relop===  const=ACC_SensorMaxDistance + 1  OutDataTypeStr=boolean
  Compare To Constant1 : simulink/Logic and Bit Operations/Compare To Constant  relop=~=  const=ACC_SensorMaxDistance + 1  OutDataTypeStr=boolean
  Compare To Zero : simulink/Logic and Bit Operations/Compare To Zero  relop===  OutDataTypeStr=boolean
  Constant : Constant  Value=15
  Detect Increase : simulink/Logic and Bit Operations/Detect Increase  vinit=0.0  OutDataTypeStr=boolean
  Detect Increase1 : simulink/Logic and Bit Operations/Detect Increase  vinit=0.0  OutDataTypeStr=boolean
  Discrete PID Controller1 : slpidlib/PID Controller  Controller=PI  Form=Parallel  TimeDomain=Discrete-time  UseExternalTs=off  SampleTime=-1  IntegratorMethod=Forward Euler  FilterMethod=Forward Euler  ControllerParametersSource=internal  P=ACC_Classic_P  I=ACC_Classic_I  UseKiTs=off  D=0  N=100  UseFilter=on  TunerSelectOption=Transfer Function Based (PID Tuner App)  InitialConditionSource=internal  InitialConditionForIntegrator=0  InitialConditionForFilter=0  DifferentiatorICPrevScaledInput=0  ExternalReset=either  TrackingMode=off  Kt=1  LimitOutput=on  SatLimitsSource=internal  UpperSaturationLimit=ACC_MaxThrottle  LowerSaturationLimit=-ACC_MaxBrake  LinearizeAsGain=off  AntiWindupMode=back-calculation  Kb=1  LimitIntegrator=off  UpperIntegratorSaturationLimit=inf  LowerIntegratorSaturationLimit=-inf  POutMin=[]  POutMax=[]  IOutMin=[]  IOutMax=[]  DOutMin=[]  DOutMax=[]  NOutMin=[]  NOutMax=[]  SumOutMin=[]  SumOutMax=[]  SaturationOutMin=[]  SaturationOutMax=[]  PParamMin=[]  PParamMax=[]  IParamMin=[]  IParamMax=[]  DParamMin=[]  DParamMax=[]  NParamMin=[]  NParamMax=[]  KbParamMin=[]  KbParamMax=[]  KtParamMin=[]  KtParamMax=[]  KbOutMin=[]  KbOutMax=[]  KtOutMin=[]  KtOutMax=[]  IntegratorOutMin=[]  IntegratorOutMax=[]  FilterOutMin=[]  FilterOutMax=[]  SumI1OutMin=[]  SumI1OutMax=[]  SumI2OutMin=[]  SumI2OutMax=[]  SumI3OutMin=[]  SumI3OutMax=[]  SumI4OutMin=[]  SumI4OutMax=[]  SumDOutMin=[]  SumDOutMax=[]  DifferentiatorOutMin=[]  DifferentiatorOutMax=[]  FilterDiffOutCoefMin=[]  FilterDiffOutCoefMax=[]  ReciprocalOutMin=[]  ReciprocalOutMax=[]  SumDenOutMin=[]  SumDenOutMax=[]  SumNumOutMin=[]  SumNumOutMax=[]  DivideOutMin=[]  DivideOutMax=[]  UdiffTsProdOutMin=[]  UdiffTsProdOutMax=[]  NTsProdOutMin=[]  NTsProdOutMax=[]  UintegralTsProdOutMin=[]  UintegralTsProdOutMax=[]  UngainTsProdOutMin=[]  UngainTsProdOutMax=[]  ClampingZeroOutDataTypeStr=Inherit: Inherit via back propagation  ClampingZeroOutMin=[]  ClampingZeroOutMax=[]  FilterDenConstantOutDataTypeStr=Inherit: Inherit via back propagation  FilterDenConstantOutMin=[]  FilterDenConstantOutMax=[]  PCopyOutDataTypeStr=Inherit: Inherit via back propagation  PCopyOutMin=[]  PCopyOutMax=[]  NCopyOutDataTypeStr=Inherit: Inherit via back propagation  NCopyOutMin=[]  NCopyOutMax=[]  IntegratorContinuousStateAttributes=''  IntegratorStateMustResolveToSignalObject=off  IntegratorRTWStateStorageClass=Auto  FilterContinuousStateAttributes=''  FilterStateMustResolveToSignalObject=off  FilterRTWStateStorageClass=Auto  ParallelPVariant=InternalParameters  IdealPVariant=Disabled  IVariant=InternalParameters  DVariant=Disabled  IntegratorVariant=Discrete  SatVariant=Enabled  AWVariant=BackCalculation  PCopyVariant=Disabled  TRVariant=Disabled  FdbkBlocksVariant=Forward  IdealPFdbkVariant=Disabled  SatFdbkVariant=Disabled  DerivativeFilterVariant=Disabled  NVariant=Disabled  NCopyVariant=Disabled_SignalSpec  FilterICVariant=Disabled  IntegratorICVariant=InternalICs  ExternalResetVariant=ExternalReset  TRSumVariant=Passthrough  SumFdbkVariant=Disabled  SumVariant=Sum_PI  TsampFilterVariant=InternalTs  TsampNgainVariant=Passthrough  TsampIntegralVariant=Passthrough  ExternalSaturationOutDataTypeStr=Inherit: Same as second input
  Error : Sum  Inputs=+-
  Error1 : Sum  Inputs=-+
  Error2 : Sum  Inputs=+-
  Memory : Memory
  Memory1 : Memory
  Memory2 : Memory
  MinMax : MinMax
  MinMax1 : MinMax
  MinMax2 : MinMax  Inputs=2
  OR : Logic  Operator=OR  AllPortsSameDT=off  OutDataTypeStr=boolean
  Product{,1..9} (10 alike) : Product
  Rate Transition : RateTransition  OutPortSampleTime=1/50
  Rate Transition1 : RateTransition  OutPortSampleTime=1/50
  Saturation1 : Saturate  UpperLimit=0  LowerLimit=-100
  Saturation2 : Saturate  UpperLimit=0  LowerLimit=-100
  Saturation3 : Saturate  UpperLimit=100  LowerLimit=0
  Saturation4 : Saturate  UpperLimit=100  LowerLimit=0
  Saturation8 : Saturate  UpperLimit=100  LowerLimit=-100
  Saturation9 : Saturate  UpperLimit=100  LowerLimit=-100
  Sum : Sum  Inputs=+++
  Sum1 : Sum  Inputs=+++
  Sum2 : Sum
  Sum3 : Sum  Inputs=-+
  Switch : Switch  Criteria=u2 > Threshold  SaturateOnIntegerOverflow=off  InputSameDT=off
  Switch1 : Switch  Criteria=u2 > Threshold  SaturateOnIntegerOverflow=off  InputSameDT=off
  Switch2 : Switch  Criteria=u2 > Threshold  SaturateOnIntegerOverflow=off  InputSameDT=off
  Target_Distance_Saturation : Saturate  UpperLimit=ACC_SensorMaxDistance  LowerLimit=2
  Terminator : Terminator
  Terminator1 : Terminator
  Terminator2 : Terminator
  Transfer Fcn First Order{4..11} (8 alike) : simulink/Discrete/Transfer Fcn First Order  PoleZ=0.9  ICPrevOutput=0.0  DoSatur=off
  Transfer Fcn First Order13 : simulink/Discrete/Transfer Fcn First Order  PoleZ=0.99  ICPrevOutput=0.0  DoSatur=off
  tACC_PID : Subsystem
  tag scope: ACC_Actual_Distance=global, ACC_Brake=global, ACC_Memory_Speed=global, ACC_PID_Output=global, ACC_Target_Distance=global, ACC_Target_Speed=global, ACC_Throttle=global, cACC_Brake_Demand=global, cACC_Throttle_Demand=global, tACC_Brake_Demand=global, tACC_PID_Output=global, tACC_Throttle_Demand=global
  wires:
  [ACC_Active] -> Product4/1
  MinMax1/1 -> Compare To Constant1/1
  Target_Distance_Saturation/1 -> [ACC_Target_Distance], Error1/1
  [Vehicle_Speed] -> Error/2
  [ACC_Active] -> Detect Increase/1, Product1/2, Product2/1
  Memory/1 -> Switch/3
  Error/1 -> Product1/1
  MinMax/1 -> Compare To Constant/1
  [SensorTargets_300000_ClosestTargetDistance] -> MinMax/1
  [Vehicle_Speed] -> Sum3/2
  Switch/1 -> Sum2/2
  Product1/1 -> ACC_PID/1  "difference betweer reference and actual speed"
  [ACC_Active] -> Compare To Zero/1
  Compare To Constant/1 -> Product2/2
  Compare To Constant1/1 -> Product4/2
  Compare To Zero/1 -> Product/2, Product5/1
  [Driver_Brake] -> Product/1
  [Driver_Throttle] -> Product5/2
  Sum1/1 -> Transfer Fcn First Order5/1
  Product5/1 -> Sum1/1
  ACC_PID/1 -> Product6/1
  Product6/1 -> Saturation2/1, Saturation3/1
  [ACC_Target_Speed] -> Error2/1
  [Vehicle_Speed] -> ACC_Speed_Distance_Gain/1(In1), Error2/2
  Saturation2/1 -> ACC_Brake_Gain1/1
  Saturation3/1 -> [cACC_Throttle_Demand]
  ACC_Brake_Gain1/1 -> [cACC_Brake_Demand]
  Product/1 -> Sum/3
  Saturation1/1 -> ACC_Brake_Gain2/1
  Saturation4/1 -> [tACC_Throttle_Demand]
  ACC_Brake_Gain2/1 -> [tACC_Brake_Demand]
  Discrete PID Controller1/1 -> Product9/1
  [cACC_Throttle_Demand] -> Sum1/2
  [cACC_Brake_Demand] -> Sum/2
  [tACC_Brake_Demand] -> Sum/1
  [tACC_Throttle_Demand] -> Sum1/3
  Product4/1 -> Product7/2, tACC_PID/2(In2), Product9/2, Discrete PID Controller1/2
  MinMax2/1 -> Saturation4/1, Saturation1/1, [tACC_PID_Output]
  Error2/1 -> Discrete PID Controller1/1
  Product9/1 -> MinMax2/1
  Product2/1 -> Product6/2, ACC_PID/2
  Transfer Fcn First Order5/1 -> Transfer Fcn First Order4/1
  Sum/1 -> Transfer Fcn First Order9/1
  Transfer Fcn First Order4/1 -> Transfer Fcn First Order6/1
  Transfer Fcn First Order6/1 -> Transfer Fcn First Order7/1
  Transfer Fcn First Order7/1 -> Saturation9/1
  Transfer Fcn First Order8/1 -> Transfer Fcn First Order10/1
  Transfer Fcn First Order9/1 -> Transfer Fcn First Order8/1
  Transfer Fcn First Order10/1 -> Transfer Fcn First Order11/1
  Transfer Fcn First Order11/1 -> Saturation8/1
  Saturation8/1 -> [ACC_Brake]
  Saturation9/1 -> [ACC_Throttle]
  Product7/1 -> MinMax2/2
  [SensorTargets_300000_ClosestTargetDistance] -> Transfer Fcn First Order13/1, MinMax1/1, Rate Transition/1
  Transfer Fcn First Order13/1 -> [ACC_Actual_Distance]
  ACC_Speed_Distance_Gain/1(Out1) -> Rate Transition1/1
  Error1/1 -> tACC_PID/1(In1)
  tACC_PID/1(Out1) -> [ACC_PID_Output], Product7/1
  [Additional_speed] -> Product3/1
  Detect Increase/1 -> Switch/2
  Product8/1 -> Switch1/3, [ACC_Target_Speed], Memory1/1
  Switch1/1 -> Memory/1, Error/1
  [reset_ACC] -> Detect Increase1/1
  [ACC_Memory_Speed] -> Switch1/1
  Detect Increase1/1 -> Switch1/2
  Rate Transition/1 -> Error1/2
  Rate Transition1/1 -> Target_Distance_Saturation/1
  Product3/1 -> Sum2/1
  ACC_Module_Activity_Flag/1 -> OR/1
  Sum2/1 -> Product8/1
  [ACC_Active] -> Product3/2
  [Driver_Throttle] -> ACC_PID/3
  [ACC_Active] -> Switch2/2
  Switch2/1 -> Memory2/1, [ACC_Memory_Speed]  "set speed memory"
  Memory1/1 -> Switch2/1
  Memory2/1 -> Switch2/3
  AP_Module_Activity_Flag/1 -> OR/2
  OR/1 -> Product8/2
  Sum3/1 -> Switch/1
  Constant/1 -> Sum3/1
  [ACC_Target_Distance] -> Terminator/1
  [ACC_Actual_Distance] -> Terminator1/1
  [ACC_PID_Output] -> Bus Creator/1
  [tACC_PID_Output] -> Bus Creator/2
  [tACC_Brake_Demand] -> Bus Creator/3
  [tACC_Throttle_Demand] -> Bus Creator/4
  Bus Creator/1 -> Terminator2/1
